simulink model "Grue_L"  (Simulink 9.2)
settings: Solver=ode4  StartTime=0.0  StopTime=20  FixedStep=1e-3  RelTol=1e-3  EnableMultiTasking=on
values from neighbouring files (symbols this model uses):
  b = 0.4    [Ini_Grue.m]
  Cd = 20    [Ini_Grue.m]
  Cr = 20    [Ini_Grue.m]    (also in plot_things.m = Cr*kc)
  eta = -1/(C_1*(A-B*K)^-1*B_1)    [Ini_Grue.m]
  g = 10    [Ini_Grue.m]
  J = 50    [Ini_Grue.m]
  K = place(A,B,p)    [Ini_Grue.m]
  m = 500    [Ini_Grue.m]    (also in plot_things.m)
  Mc = 5000    [Ini_Grue.m]
  R = 15    [Ini_Grue.m]
  Ti = 5e-4    (= 0.0005)    [plot_things.m]
settings Model: Creator=abbasturki  LastModifiedBy=pac
settings OptimizationCC: ExpressionDepthLimit=2147483647
settings DebuggingCC: SolverPrmCheckMsg=warning

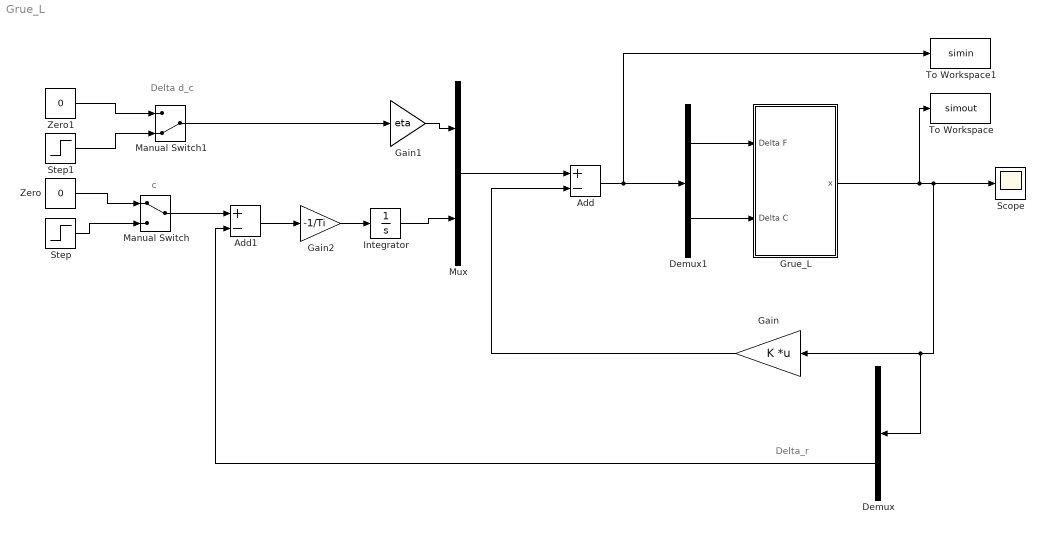
== system Grue_L ==
  note: c
  note: Delta d_c
  note: Delta_r
  Add : Sum  Inputs=+-
  Add1 : Sum  Inputs=+-
  Demux : Demux  Outputs=6
  Demux1 : Demux  Outputs=2
  Gain : Gain  Gain=K  Multiplication=Matrix(K*u) (u vector)
  Gain1 : Gain  Gain=eta
  Gain2 : Gain  Gain=-1/Ti
  Grue_L : Subsystem
  Integrator : Integrator
  Manual Switch : ManualSwitch
  Manual Switch1 : ManualSwitch  CurrentSetting=0
  Mux : Mux  Inputs=2
  Scope : Scope
  Step : Step  SampleTime=0
  Step1 : Step  After=20  SampleTime=0
  To Workspace : ToWorkspace  VariableName=simout  SaveFormat=Timeseries  SampleTime=-1
  To Workspace1 : ToWorkspace  VariableName=simin  SaveFormat=Timeseries  SampleTime=-1
  Zero : Constant  Value=0  OutDataTypeStr=Inherit: Inherit via back propagation
  Zero1 : Constant  Value=0  OutDataTypeStr=Inherit: Inherit via back propagation
  wires:
  Demux1/1 -> Grue_L/1(Delta F)
  Demux1/2 -> Grue_L/2(Delta C)
  Gain/1 -> Add/2
  Add/1 -> To Workspace1/1, Demux1/1
  Mux/1 -> Add/1
  Gain1/1 -> Mux/1
  Grue_L/1(x) -> To Workspace/1, Demux/1, Gain/1, Scope/1
  Gain2/1 -> Integrator/1
  Integrator/1 -> Mux/2
  Add1/1 -> Gain2/1
  Demux/5 -> Add1/2
  Step/1 -> Manual Switch/2
  Manual Switch/1 -> Add1/1
  Zero/1 -> Manual Switch/1
  Manual Switch1/1 -> Gain1/1
  Zero1/1 -> Manual Switch1/1
  Step1/1 -> Manual Switch1/2

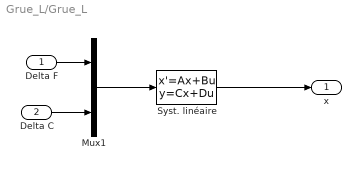
== system Grue_L/Grue_L ==
  Delta F : Inport
  Delta C : Inport  Port=2
  Mux1 : Mux  Inputs=2
  Syst. linéaire : StateSpace  A=[0 0 0 1 0 0 ; 0 0 0 0 1 0 ; 0 0 0 0 0 1 ; 0 0 m*g/Mc -Cd/Mc 0 0 ; 0 0 0 0 -Cr/(b^2*(J/b^2+m)) 0 ; 0 0 -g/R*(1+m/Mc) Cd/(Mc*R) 0 0]  B=[0 0 ; 0 0 ; 0 0 ; 1/Mc 0 ; 0 -1/(b*(J/b^2+m)) ; -1/(R*Mc) 0 ];  C=eye(6)  D=zeros(6,2)  InitialCondition=0
  x : Outport
  wires:
  Mux1/1 -> Syst. linéaire/1
  Delta F/1 -> Mux1/1
  Delta C/1 -> Mux1/2
  Syst. linéaire/1 -> x/1
